simulink model "get_hoops"  (R2022a)
settings: Solver=VariableStepAuto  StartTime=0.0  StopTime=10.0  RelTol=1e-3
libraries: robotlib x4
settings Model: Creator=dtu31390  LastModifiedBy=dtu31390

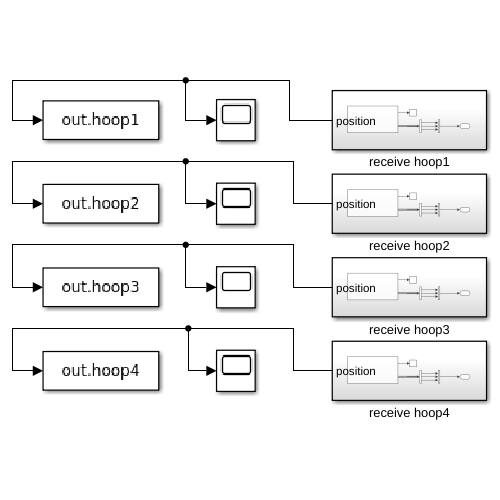
[thumbnail: Simulink's stored preview of the top-level diagram]
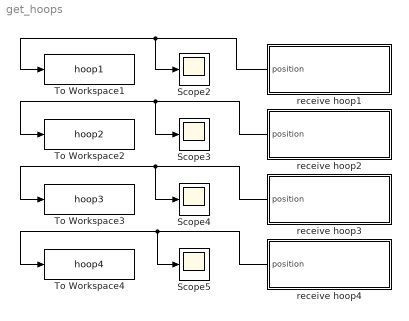
== system get_hoops ==
  Scope{2..5} (4 alike) : Scope
  To Workspace1 : ToWorkspace  VariableName=hoop1  SaveFormat=Timeseries  SampleTime=-1
  To Workspace2 : ToWorkspace  VariableName=hoop2  SaveFormat=Timeseries  SampleTime=-1
  To Workspace3 : ToWorkspace  VariableName=hoop3  SaveFormat=Timeseries  SampleTime=-1
  To Workspace4 : ToWorkspace  VariableName=hoop4  SaveFormat=Timeseries  SampleTime=-1
  receive hoop1 : Subsystem
  receive hoop2 : Subsystem
  receive hoop3 : Subsystem
  receive hoop4 : Subsystem
  wires:
  receive hoop1/1(position) -> To Workspace1/1, Scope2/1
  receive hoop3/1(position) -> Scope4/1, To Workspace3/1
  receive hoop2/1(position) -> To Workspace2/1, Scope3/1
  receive hoop4/1(position) -> To Workspace4/1, Scope5/1

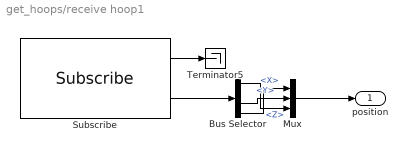
== system get_hoops/receive hoop1 ==
  Bus Selector : BusSelector  OutputSignals=Pose.Position.Z,Pose.Position.Z,Pose.Position.Y,Pose.Position.X
  Mux : Mux  Inputs=3
  Subscribe : robotlib/Subscribe  topicSource=Select from ROS network  topic=/vrpn_client_node/hoop1/pose  messageType=geometry_msgs/PoseStamped  SampleTime=-1  legacyBusStruct=off  messageQueueLength=1
  Terminator5 : Terminator
  position : Outport
  wires:
  Subscribe/2 -> Bus Selector/1
  Mux/1 -> position/1
  Bus Selector/1 -> Mux/3  "<Z>"
  Bus Selector/4 -> Mux/1  "<X>"
  Bus Selector/3 -> Mux/2  "<Y>"
  Subscribe/1 -> Terminator5/1

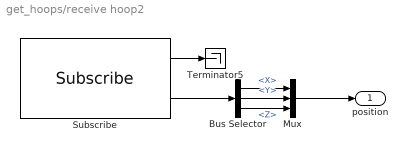
== system get_hoops/receive hoop2 ==
  Bus Selector : BusSelector  OutputSignals=Pose.Position.X,Pose.Position.Y,Pose.Position.Z
  Mux : Mux  Inputs=3
  Subscribe : robotlib/Subscribe  topicSource=Select from ROS network  topic=/vrpn_client_node/hoop2/pose  messageType=geometry_msgs/PoseStamped  SampleTime=-1  legacyBusStruct=off  messageQueueLength=1
  Terminator5 : Terminator
  position : Outport
  wires:
  Subscribe/2 -> Bus Selector/1
  Mux/1 -> position/1
  Bus Selector/3 -> Mux/3  "<Z>"
  Bus Selector/1 -> Mux/1  "<X>"
  Bus Selector/2 -> Mux/2  "<Y>"
  Subscribe/1 -> Terminator5/1

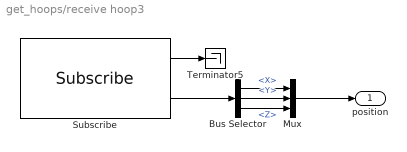
== system get_hoops/receive hoop3 ==
  Bus Selector : BusSelector  OutputSignals=Pose.Position.X,Pose.Position.Y,Pose.Position.Z
  Mux : Mux  Inputs=3
  Subscribe : robotlib/Subscribe  topicSource=Select from ROS network  topic=/vrpn_client_node/hoop3/pose  messageType=geometry_msgs/PoseStamped  SampleTime=-1  legacyBusStruct=off  messageQueueLength=1
  Terminator5 : Terminator
  position : Outport
  wires:
  Subscribe/2 -> Bus Selector/1
  Mux/1 -> position/1
  Bus Selector/3 -> Mux/3  "<Z>"
  Bus Selector/1 -> Mux/1  "<X>"
  Bus Selector/2 -> Mux/2  "<Y>"
  Subscribe/1 -> Terminator5/1

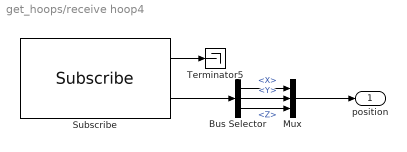
== system get_hoops/receive hoop4 ==
  Bus Selector : BusSelector  OutputSignals=Pose.Position.X,Pose.Position.Y,Pose.Position.Z
  Mux : Mux  Inputs=3
  Subscribe : robotlib/Subscribe  topicSource=Select from ROS network  topic=/vrpn_client_node/hoop4/pose  messageType=geometry_msgs/PoseStamped  SampleTime=-1  legacyBusStruct=off  messageQueueLength=1
  Terminator5 : Terminator
  position : Outport
  wires:
  Subscribe/2 -> Bus Selector/1
  Mux/1 -> position/1
  Bus Selector/3 -> Mux/3  "<Z>"
  Bus Selector/1 -> Mux/1  "<X>"
  Bus Selector/2 -> Mux/2  "<Y>"
  Subscribe/1 -> Terminator5/1
